simulink model "SmallAerobaticAirplaneModel_Simulink"  (R2018a)
settings: Solver=FixedStepAuto  StartTime=0.0  StopTime=tf  FixedStep=dt  RelTol=1e-3
values from neighbouring files (symbols this model uses):
  ail_lwr_lim = -25.2    [airplane_ic_constants.m]
  ail_upr_lim = 25.2    [airplane_ic_constants.m]
  airDensityBreakpoints = (-5:5:40)*10^3    [airplane_ic_constants.m]
  airDensityData = [27.45, 23.77, 20.48, 17.56, 14.96, 12.67, 10.66, 8.91, 7.38, 5.87]*10^(-4)    [airplane_ic_constants.m]
  elev_lwr_lim = -17.2    [airplane_ic_constants.m]
  elev_upr_lim = 17.2    [airplane_ic_constants.m]
  mass = weight/32.17    (= 0.901460988499)    [airplane_ic_constants.m]
  rud_lwr_lim = -28.65    [airplane_ic_constants.m]
  rud_upr_lim = 28.65    [airplane_ic_constants.m]
  weight = 29    [airplane_ic_constants.m]
  Xfuse = -1.5    [airplane_ic_constants.m]
  Xfuse_uu = 0.15    [airplane_ic_constants.m]
  Xht = -3.5    [airplane_ic_constants.m]
  Xp = 2.2    [airplane_ic_constants.m]
  Xvt = -4.1    [airplane_ic_constants.m]
  Xw = 0.2    [airplane_ic_constants.m]
  Yfuse_vv = 1.2    [airplane_ic_constants.m]
  Yht = 0    [airplane_ic_constants.m]
  Yvt = 0    [airplane_ic_constants.m]
  Yw = 2.0    (= 2)    [airplane_ic_constants.m]
  Zfuse = 0    [airplane_ic_constants.m]
  Zfuse_ww = 1.0    (= 1)    [airplane_ic_constants.m]
  Zht = 0    [airplane_ic_constants.m]
  Zp = 0    [airplane_ic_constants.m]
  Zvt = -0.60    (= -0.6)    [airplane_ic_constants.m]
  Zw = 0    [airplane_ic_constants.m]
settings Model: Creator=Kyle  LastModifiedBy=Kyle
settings DataIOCC: LoadExternalInput=on

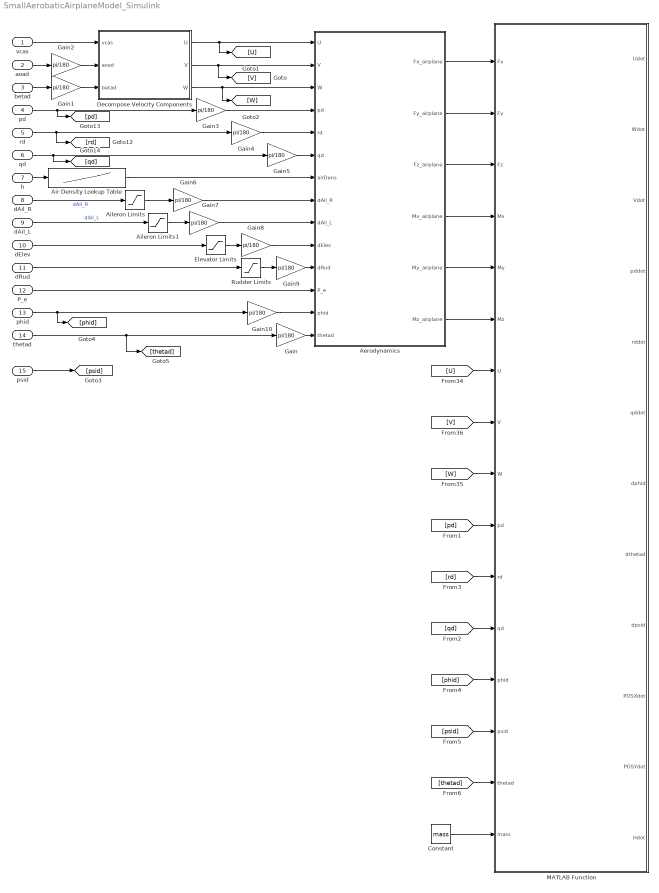
== system SmallAerobaticAirplaneModel_Simulink ==
  vcas : Inport
  aoad : Inport  Port=2
  betad : Inport  Port=3
  pd : Inport  Port=4
  rd : Inport  Port=5
  qd : Inport  Port=6
  h : Inport  Port=7
  dAil_R : Inport  Port=8
  dAil_L : Inport  Port=9
  dElev : Inport  Port=10
  dRud : Inport  Port=11
  P_e : Inport  Port=12
  phid : Inport  Port=13
  thetad : Inport  Port=14
  psid : Inport  Port=15
  Aerodynamics : Subsystem
  Aileron Limits : Saturate  UpperLimit=ail_upr_lim  LowerLimit=ail_lwr_lim
  Aileron Limits1 : Saturate  UpperLimit=ail_upr_lim  LowerLimit=ail_lwr_lim
  Air Density Lookup Table : Lookup_n-D  NumberOfTableDimensions=1  BreakpointsForDimension1=airDensityBreakpoints  Table=airDensityData  InternalRulePriority=Speed  RndMeth=Simplest  InputSameDT=on
  Constant : Constant  Value=mass
  Decompose Velocity Components : Subsystem
  Elevator Limits : Saturate  UpperLimit=elev_upr_lim  LowerLimit=elev_lwr_lim
  Gain{,1..10} (11 alike) : Gain  Gain=pi/180
  MATLAB Function : MATLAB Function  TreatAsAtomicUnit=on
  Rudder Limits : Saturate  UpperLimit=rud_upr_lim  LowerLimit=rud_lwr_lim
  wires:
  h/1 -> Air Density Lookup Table/1
  vcas/1 -> Decompose Velocity Components/1(vcas)
  aoad/1 -> Gain2/1
  betad/1 -> Gain1/1
  Decompose Velocity Components/1(U) -> [U], Aerodynamics/1(U)
  Decompose Velocity Components/2(V) -> [V], Aerodynamics/2(V)
  Decompose Velocity Components/3(W) -> [W], Aerodynamics/3(W)
  pd/1 -> [pd], Gain3/1
  rd/1 -> [rd], Gain4/1
  qd/1 -> [qd], Gain5/1
  Air Density Lookup Table/1 -> Aerodynamics/7(airDens)
  dElev/1 -> Elevator Limits/1
  P_e/1 -> Aerodynamics/12(P_e)
  phid/1 -> [phid], Gain10/1
  thetad/1 -> [thetad], Gain/1
  Gain/1 -> Aerodynamics/14(thetad)
  Gain1/1 -> Decompose Velocity Components/3(betad)
  Gain2/1 -> Decompose Velocity Components/2(aoad)
  Gain3/1 -> Aerodynamics/4(pd)
  Gain4/1 -> Aerodynamics/5(rd)
  Gain5/1 -> Aerodynamics/6(qd)
  Aileron Limits1/1 -> Gain7/1
  Gain9/1 -> Aerodynamics/11(dRud)
  Rudder Limits/1 -> Gain9/1
  dRud/1 -> Rudder Limits/1
  Gain8/1 -> Aerodynamics/10(dElev)
  Elevator Limits/1 -> Gain8/1
  Gain7/1 -> Aerodynamics/9(dAil_L)
  dAil_L/1 -> Aileron Limits1/1  "dAil_L"
  Aileron Limits/1 -> Gain6/1
  Gain6/1 -> Aerodynamics/8(dAil_R)
  dAil_R/1 -> Aileron Limits/1  "dAil_R"
  Aerodynamics/1(Fx_airplane) -> MATLAB Function/1(Fx)
  Aerodynamics/2(Fy_airplane) -> MATLAB Function/2(Fy)
  Aerodynamics/3(Fz_airplane) -> MATLAB Function/3(Fz)
  Aerodynamics/4(Mx_airplane) -> MATLAB Function/4(Mx)
  Aerodynamics/5(My_airplane) -> MATLAB Function/5(My)
  Aerodynamics/6(Mz_airplane) -> MATLAB Function/6(Mz)
  [U] -> MATLAB Function/7(U)
  [V] -> MATLAB Function/8(V)
  [W] -> MATLAB Function/9(W)
  [qd] -> MATLAB Function/12(qd)
  [rd] -> MATLAB Function/11(rd)
  [pd] -> MATLAB Function/10(pd)
  Gain10/1 -> Aerodynamics/13(phid)
  [phid] -> MATLAB Function/13(phid)
  [psid] -> MATLAB Function/14(psid)
  [thetad] -> MATLAB Function/15(thetad)
  Constant/1 -> MATLAB Function/16(mass)
  psid/1 -> [psid]

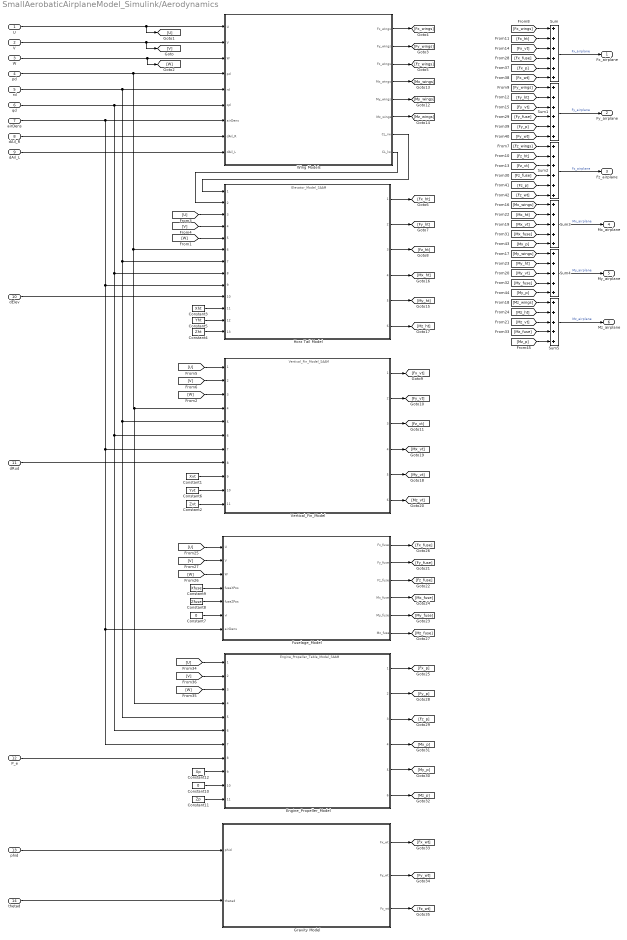
== system SmallAerobaticAirplaneModel_Simulink/Aerodynamics ==
  U : Inport
  V : Inport  Port=2
  W : Inport  Port=3
  pd : Inport  Port=4
  rd : Inport  Port=5
  qd : Inport  Port=6
  airDens : Inport  Port=7
  dAil_R : Inport  Port=8
  dAil_L : Inport  Port=9
  dElev : Inport  Port=10
  dRud : Inport  Port=11
  P_e : Inport  Port=12
  phid : Inport  Port=13
  thetad : Inport  Port=14
  Constant1 : Constant  Value=Xvt
  Constant10 : Constant  Value=0
  Constant11 : Constant  Value=Zp
  Constant12 : Constant  Value=Xp
  Constant2 : Constant  Value=Zvt
  Constant3 : Constant  Value=Xht
  Constant4 : Constant  Value=Zht
  Constant5 : Constant  Value=Yht
  Constant6 : Constant  Value=Yvt
  Constant7 : Constant  Value=0
  Constant8 : Constant  Value=Zfuse
  Constant9 : Constant  Value=Xfuse
  Engine_Propeller_Model : ModelReference  ModelNameDialog=Engine_Propeller_Table_Model_SAAM.slx  SimulationMode=Normal  ModelReferenceVersion=1.93
  Fuselage_Model : Subsystem
  Gravity Model : Subsystem
  Horz Tail Model : ModelReference  ModelNameDialog=Elevator_Model_SAAM.slx  SimulationMode=Normal  ModelReferenceVersion=1.31
  Sum : Sum  Inputs=++++++
  Sum1 : Sum  Inputs=++++++
  Sum2 : Sum  Inputs=++++++
  Sum3 : Sum  Inputs=+++++
  Sum4 : Sum  Inputs=+++++
  Sum5 : Sum  Inputs=+++++
  Vertical_Fin_Model : ModelReference  ModelNameDialog=Vertical_Fin_Model_SAAM.slx  SimulationMode=Normal  ModelReferenceVersion=1.46
  Wing Models : Subsystem
  Fx_airplane : Outport
  Fy_airplane : Outport  Port=2
  Fz_airplane : Outport  Port=3
  Mx_airplane : Outport  Port=4
  My_airplane : Outport  Port=5
  Mz_airplane : Outport  Port=6
  wires:
  Gravity Model/1(Fx_wt) -> [Fx_wt]
  [Mx_p] -> Sum3/5
  [Mx_fuse] -> Sum3/4
  Gravity Model/3(Fz_wt) -> [Fz_wt]
  [Fy_wt] -> Sum1/6
  Horz Tail Model/6 -> [Mz_ht]
  Sum3/1 -> Mx_airplane/1  "Mx_airplane"
  pd/1 -> Engine_Propeller_Model/4, Vertical_Fin_Model/4, Horz Tail Model/6, Wing Models/4(pd)
  Constant9/1 -> Fuselage_Model/4(fuseXPos)
  [Fy_p] -> Sum1/5
  P_e/1 -> Engine_Propeller_Model/8
  [Fz_wings] -> Sum2/1
  [Mz_vt] -> Sum5/3
  [Fz_p] -> Sum2/5
  [Fy_vt] -> Sum1/3
  [Fx_wings] -> Sum/1
  airDens/1 -> Engine_Propeller_Model/7, Fuselage_Model/7(airDens), Vertical_Fin_Model/7, Horz Tail Model/9, Wing Models/7(airDens)
  U/1 -> [U], Wing Models/1(U)
  Horz Tail Model/3 -> [Fz_ht]
  [My_p] -> Sum4/5
  [V] -> Vertical_Fin_Model/2
  [Fx_p] -> Sum/5
  [Mx_wings] -> Sum3/1
  Vertical_Fin_Model/5 -> [My_vt]
  [Fy_ht] -> Sum1/2
  Sum2/1 -> Fz_airplane/1  "Fz_airplane"
  qd/1 -> Engine_Propeller_Model/6, Vertical_Fin_Model/6, Horz Tail Model/8, Wing Models/6(qd)
  [Mz_wings] -> Sum5/1
  Vertical_Fin_Model/6 -> [Mz_vt]
  Constant5/1 -> Horz Tail Model/12
  [My_ht] -> Sum4/2
  rd/1 -> Engine_Propeller_Model/5, Vertical_Fin_Model/5, Horz Tail Model/7, Wing Models/5(rd)
  [Fx_wt] -> Sum/6
  [V] -> Fuselage_Model/2(V)
  Constant2/1 -> Vertical_Fin_Model/11
  [Mz_p] -> Sum5/5
  Wing Models/8(CL_lw) -> Horz Tail Model/2
  Constant7/1 -> Fuselage_Model/6(vi)
  Wing Models/6(Mz_wings) -> [Mz_wings]
  [Fz_vt] -> Sum2/3
  [Fz_wt] -> Sum2/6
  [Mx_ht] -> Sum3/2
  [Fx_vt] -> Sum/3
  Constant4/1 -> Horz Tail Model/13
  Vertical_Fin_Model/2 -> [Fy_vt]
  dRud/1 -> Vertical_Fin_Model/8
  Horz Tail Model/5 -> [My_ht]
  Wing Models/4(Mx_wings) -> [Mx_wings]
  Horz Tail Model/2 -> [Fy_ht]
  Constant1/1 -> Vertical_Fin_Model/9
  Vertical_Fin_Model/1 -> [Fx_vt]
  Wing Models/3(Fz_wings) -> [Fz_wings]
  Vertical_Fin_Model/3 -> [Fz_vt]
  Wing Models/2(Fy_wings) -> [Fy_wings]
  Constant10/1 -> Engine_Propeller_Model/10
  [Fz_ht] -> Sum2/2
  [My_vt] -> Sum4/3
  [Mz_ht] -> Sum5/2
  Horz Tail Model/1 -> [Fx_ht]
  [Fx_ht] -> Sum/2
  [My_wings] -> Sum4/1
  Wing Models/5(My_wings) -> [My_wings]
  [W] -> Fuselage_Model/3(W)
  Fuselage_Model/1(Fx_fuse) -> [Fx_fuse]
  Fuselage_Model/3(Fz_fuse) -> [Fz_fuse]
  [W] -> Horz Tail Model/5
  Constant6/1 -> Vertical_Fin_Model/10
  Fuselage_Model/2(Fy_fuse) -> [Fy_fuse]
  Fuselage_Model/5(My_fuse) -> [My_fuse]
  Fuselage_Model/4(Mx_fuse) -> [Mx_fuse]
  [Mx_vt] -> Sum3/3
  [U] -> Horz Tail Model/3
  V/1 -> [V], Wing Models/2(V)
  dElev/1 -> Horz Tail Model/10
  [Fy_fuse] -> Sum1/4
  Constant8/1 -> Fuselage_Model/5(fuseZPos)
  W/1 -> [W], Wing Models/3(W)
  [Mz_fuse] -> Sum5/4
  [W] -> Engine_Propeller_Model/3
  [V] -> Horz Tail Model/4
  Sum5/1 -> Mz_airplane/1  "Mz_airplane"
  Constant12/1 -> Engine_Propeller_Model/9
  [U] -> Fuselage_Model/1(U)
  [My_fuse] -> Sum4/4
  Constant3/1 -> Horz Tail Model/11
  [V] -> Engine_Propeller_Model/2
  Vertical_Fin_Model/4 -> [Mx_vt]
  Constant11/1 -> Engine_Propeller_Model/11
  Engine_Propeller_Model/2 -> [Fy_p]
  Engine_Propeller_Model/3 -> [Fz_p]
  [U] -> Vertical_Fin_Model/1
  Sum1/1 -> Fy_airplane/1  "Fy_airplane"
  [W] -> Vertical_Fin_Model/3
  [Fz_fuse] -> Sum2/4
  Engine_Propeller_Model/4 -> [Mx_p]
  Engine_Propeller_Model/1 -> [Fx_p]
  Engine_Propeller_Model/6 -> [Mz_p]
  Engine_Propeller_Model/5 -> [My_p]
  Gravity Model/2(Fy_wt) -> [Fy_wt]
  [U] -> Engine_Propeller_Model/1
  Wing Models/1(Fx_wings) -> [Fx_wings]
  [Fy_wings] -> Sum1/1
  Wing Models/7(CL_rw) -> Horz Tail Model/1
  Horz Tail Model/4 -> [Mx_ht]
  [Fx_fuse] -> Sum/4
  Fuselage_Model/6(Mz_fuse) -> [Mz_fuse]
  phid/1 -> Gravity Model/1(phid)
  thetad/1 -> Gravity Model/2(thetad)
  Sum4/1 -> My_airplane/1  "My_airplane"
  Sum/1 -> Fx_airplane/1  "Fx_airplane"
  dAil_R/1 -> Wing Models/8(dAil_R)
  dAil_L/1 -> Wing Models/9(dAil_L)

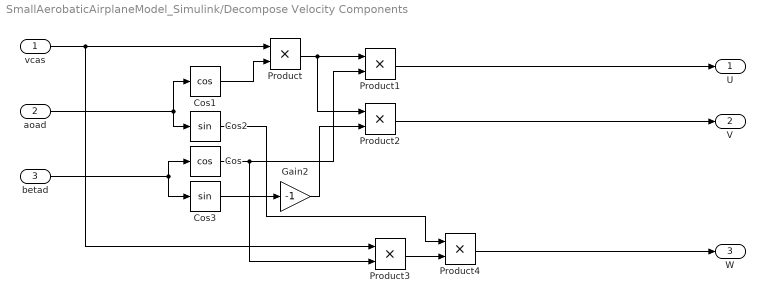
== system SmallAerobaticAirplaneModel_Simulink/Decompose Velocity Components ==
  vcas : Inport
  aoad : Inport  Port=2
  betad : Inport  Port=3
  Cos : Trigonometry  Operator=cos
  Cos1 : Trigonometry  Operator=cos
  Cos2 : Trigonometry
  Cos3 : Trigonometry
  Gain2 : Gain  Gain=-1
  Product{,1..4} (5 alike) : Product
  U : Outport
  V : Outport  Port=2
  W : Outport  Port=3
  wires:
  aoad/1 -> Cos1/1, Cos2/1
  Cos1/1 -> Product/2
  Product/1 -> Product2/1, Product1/1
  Cos2/1 -> Product4/1
  Cos/1 -> Product3/2, Product1/2
  betad/1 -> Cos3/1, Cos/1
  vcas/1 -> Product3/1, Product/1
  Product3/1 -> Product4/2
  Product2/1 -> V/1
  Cos3/1 -> Gain2/1
  Product1/1 -> U/1
  Product4/1 -> W/1
  Gain2/1 -> Product2/2

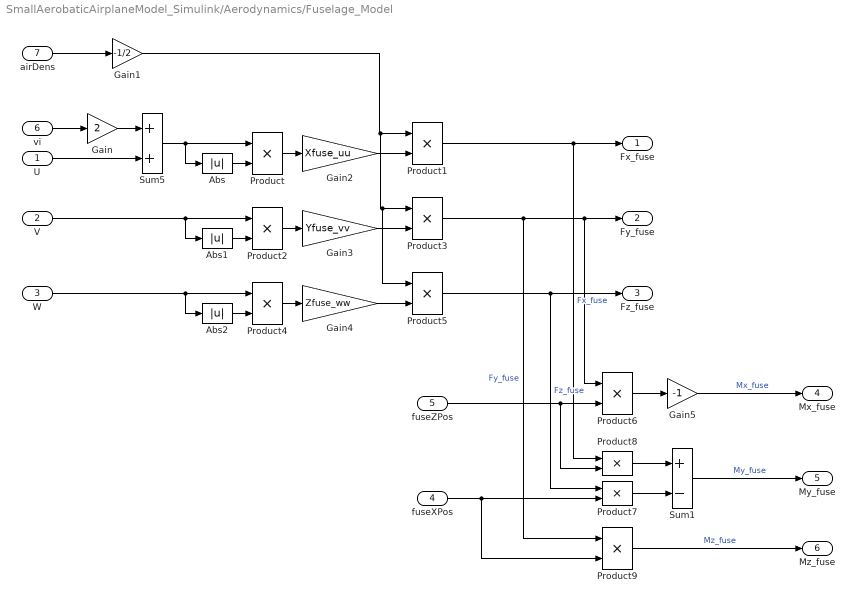
== system SmallAerobaticAirplaneModel_Simulink/Aerodynamics/Fuselage_Model ==
  U : Inport
  V : Inport  Port=2
  W : Inport  Port=3
  fuseXPos : Inport  Port=4
  fuseZPos : Inport  Port=5
  vi : Inport  Port=6
  airDens : Inport  Port=7
  Abs : Abs
  Abs1 : Abs
  Abs2 : Abs
  Gain : Gain  Gain=2
  Gain1 : Gain  Gain=-1/2
  Gain2 : Gain  Gain=Xfuse_uu
  Gain3 : Gain  Gain=Yfuse_vv
  Gain4 : Gain  Gain=Zfuse_ww
  Gain5 : Gain  Gain=-1
  Product{,1..9} (10 alike) : Product
  Sum1 : Sum  Inputs=+-
  Sum5 : Sum
  Fx_fuse : Outport
  Fy_fuse : Outport  Port=2
  Fz_fuse : Outport  Port=3
  Mx_fuse : Outport  Port=4
  My_fuse : Outport  Port=5
  Mz_fuse : Outport  Port=6
  wires:
  vi/1 -> Gain/1
  Gain/1 -> Sum5/1
  U/1 -> Sum5/2
  airDens/1 -> Gain1/1
  Sum5/1 -> Abs/1, Product/1
  Abs/1 -> Product/2
  Product/1 -> Gain2/1
  Product1/1 -> Product8/1, Fx_fuse/1  "Fx_fuse"
  Gain2/1 -> Product1/2
  V/1 -> Abs1/1, Product2/1
  Product2/1 -> Gain3/1
  Abs1/1 -> Product2/2
  Product3/1 -> Product9/1, Product6/1, Fy_fuse/1  "Fy_fuse"
  Gain3/1 -> Product3/2
  Product5/1 -> Product7/1, Fz_fuse/1  "Fz_fuse"
  Gain1/1 -> Product5/1, Product3/1, Product1/1
  Abs2/1 -> Product4/2
  Gain4/1 -> Product5/2
  Product4/1 -> Gain4/1
  W/1 -> Abs2/1, Product4/1
  Sum1/1 -> My_fuse/1  "My_fuse"
  Product9/1 -> Mz_fuse/1  "Mz_fuse"
  Product6/1 -> Gain5/1
  Gain5/1 -> Mx_fuse/1  "Mx_fuse"
  fuseZPos/1 -> Product8/2, Product6/2
  Product8/1 -> Sum1/1
  Product7/1 -> Sum1/2
  fuseXPos/1 -> Product9/2, Product7/2

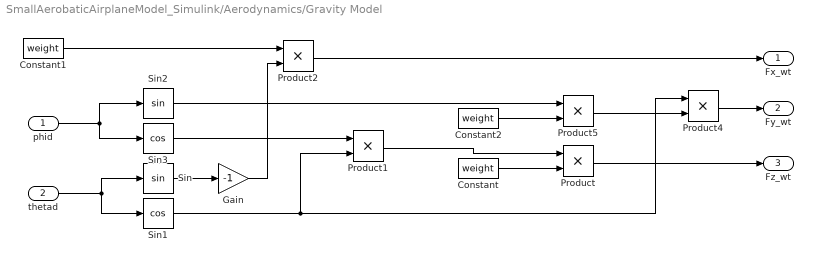
== system SmallAerobaticAirplaneModel_Simulink/Aerodynamics/Gravity Model ==
  phid : Inport
  thetad : Inport  Port=2
  Constant : Constant  Value=weight
  Constant1 : Constant  Value=weight
  Constant2 : Constant  Value=weight
  Gain : Gain  Gain=-1
  Product{,1..2,4..5} (5 alike) : Product
  Sin : Trigonometry
  Sin1 : Trigonometry  Operator=cos
  Sin2 : Trigonometry
  Sin3 : Trigonometry  Operator=cos
  Fx_wt : Outport
  Fy_wt : Outport  Port=2
  Fz_wt : Outport  Port=3
  wires:
  thetad/1 -> Sin/1, Sin1/1
  phid/1 -> Sin3/1, Sin2/1
  Sin1/1 -> Product1/2, Product4/1
  Sin/1 -> Gain/1
  Constant1/1 -> Product2/1
  Gain/1 -> Product2/2
  Product4/1 -> Fy_wt/1
  Product5/1 -> Product4/2
  Constant2/1 -> Product5/2
  Sin2/1 -> Product5/1
  Product2/1 -> Fx_wt/1
  Sin3/1 -> Product1/1
  Product/1 -> Fz_wt/1
  Product1/1 -> Product/1
  Constant/1 -> Product/2

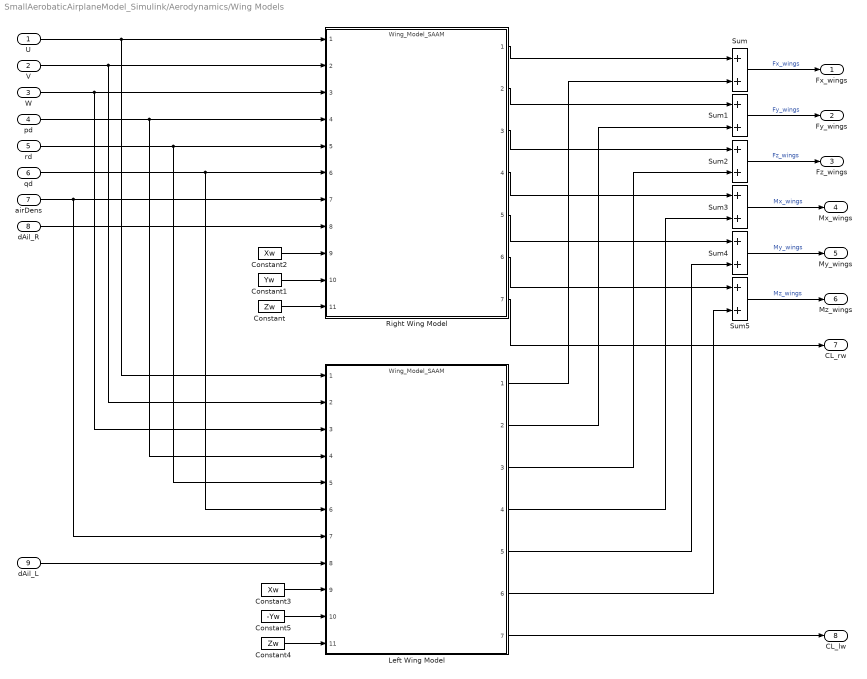
== system SmallAerobaticAirplaneModel_Simulink/Aerodynamics/Wing Models ==
  U : Inport
  V : Inport  Port=2
  W : Inport  Port=3
  pd : Inport  Port=4
  rd : Inport  Port=5
  qd : Inport  Port=6
  airDens : Inport  Port=7
  dAil_R : Inport  Port=8
  dAil_L : Inport  Port=9
  Constant : Constant  Value=Zw
  Constant1 : Constant  Value=Yw
  Constant2 : Constant  Value=Xw
  Constant3 : Constant  Value=Xw
  Constant4 : Constant  Value=Zw
  Constant5 : Constant  Value=-Yw
  Left Wing Model : ModelReference  ModelNameDialog=Wing_Model_SAAM.slx  SimulationMode=Normal  ModelReferenceVersion=1.25
  Right Wing Model : ModelReference  ModelNameDialog=Wing_Model_SAAM.slx  SimulationMode=Normal  ModelReferenceVersion=1.25
  Sum{,1..5} (6 alike) : Sum
  Fx_wings : Outport
  Fy_wings : Outport  Port=2
  Fz_wings : Outport  Port=3
  Mx_wings : Outport  Port=4
  My_wings : Outport  Port=5
  Mz_wings : Outport  Port=6
  CL_rw : Outport  Port=7
  CL_lw : Outport  Port=8
  wires:
  V/1 -> Left Wing Model/2, Right Wing Model/2
  Left Wing Model/3 -> Sum2/2
  pd/1 -> Left Wing Model/4, Right Wing Model/4
  Constant2/1 -> Right Wing Model/9
  Constant5/1 -> Left Wing Model/10
  Sum4/1 -> My_wings/1  "My_wings"
  dAil_R/1 -> Right Wing Model/8
  Constant/1 -> Right Wing Model/11
  Constant1/1 -> Right Wing Model/10
  U/1 -> Left Wing Model/1, Right Wing Model/1
  Left Wing Model/5 -> Sum4/2
  Left Wing Model/6 -> Sum5/2
  Right Wing Model/3 -> Sum2/1
  rd/1 -> Right Wing Model/5, Left Wing Model/5
  Sum1/1 -> Fy_wings/1  "Fy_wings"
  Constant3/1 -> Left Wing Model/9
  Constant4/1 -> Left Wing Model/11
  Sum/1 -> Fx_wings/1  "Fx_wings"
  Right Wing Model/2 -> Sum1/1
  Right Wing Model/5 -> Sum4/1
  Right Wing Model/1 -> Sum/1
  Sum3/1 -> Mx_wings/1  "Mx_wings"
  airDens/1 -> Left Wing Model/7, Right Wing Model/7
  Left Wing Model/2 -> Sum1/2
  W/1 -> Left Wing Model/3, Right Wing Model/3
  Right Wing Model/4 -> Sum3/1
  qd/1 -> Right Wing Model/6, Left Wing Model/6
  dAil_L/1 -> Left Wing Model/8
  Right Wing Model/6 -> Sum5/1
  Left Wing Model/1 -> Sum/2
  Left Wing Model/4 -> Sum3/2
  Sum2/1 -> Fz_wings/1  "Fz_wings"
  Sum5/1 -> Mz_wings/1  "Mz_wings"
  Left Wing Model/7 -> CL_lw/1
  Right Wing Model/7 -> CL_rw/1

== matlab function SmallAerobaticAirplaneModel_Simulink/MATLAB Function ==
  data: Fx input double size=1; Udot output double size=1; Fy input double size=1; Fz input double size=1; Mx input double size=1; My input double size=1; Mz input double size=1; U input double size=1; Wdot output double size=1; Vdot output double size=1; pddot output; rddot output double size=1; V input double size=1; qddot output; dphid output; dthetad output; W input; pd input; rd input; qd input; phid input; psid input; thetad input; mass input; dpsid output; POSXdot output; POSYdot output; Hdot output
function [Udot, Wdot, Vdot, pddot, rddot, qddot, dphid, dthetad, dpsid, POSXdot, POSYdot, Hdot] = ForceToDeriv(Fx, Fy, Fz, Mx, My, Mz, U, V, W, pd, rd, qd, phid, psid, thetad, mass)
%UNTITLED Summary of this function goes here
%   Detailed explanation goes here

Jx = 0.32;
Jy = 1.5;
Jz = 2.3;

D2R = pi/180;

PHI = phid*D2R;
PSI = psid*D2R;
THETA = thetad*D2R;

P = pd*D2R;
R = rd*D2R;
Q = qd*D2R;

Udot = R*V - Q*W + Fx/mass;
Vdot = P*W - R*U + Fy/mass;
Wdot = Q*U - P*V + Fz/mass;

Pdot = (Mx + (Jy-Jz)*R*Q) / Jx;
Rdot = (My + (Jz-Jx)*P*Q) / Jy;
Qdot = (Mz + (Jx-Jy)*R*P) / Jz;

PHIdot = P + Q*sin(PHI)*tan(THETA) + cos(PHI)*tan(THETA);
THETAdot = Q*cos(PHI) - R*sin(PHI);
PSIdot = ( Q*sin(PHI) - R*cos(PHI) ) / min(0.001,cos(THETA));

Te2b = [cos(PSI)*cos(PHI),                              sin(PSI)*cos(PHI),                              -sin(PHI);
        cos(PSI)*sin(THETA)*sin(PHI)-sin(PSI)*cos(PHI), sin(PSI)*sin(THETA)*sin(PHI)+cos(PSI)*cos(PHI), cos(THETA)*sin(PHI);
        cos(PSI)*sin(THETA)*cos(PHI)-sin(PSI)*sin(PHI), sin(PSI)*sin(THETA)*cos(PHI)+cos(PSI)*sin(PHI), cos(THETA)*cos(PHI)];

POSdot = [U, V, W]*Te2b;

pddot = Pdot/D2R;
rddot = Rdot/D2R;
qddot = Qdot/D2R;

dphid = PHIdot/D2R;
dthetad = THETAdot/D2R;
dpsid = PSIdot/D2R;

POSXdot = POSdot(1);
POSYdot = POSdot(2);
Hdot = -POSdot(3);



end
